simulink model "EDDA_1st"  (R2020a)
settings: Solver=ode45  StartTime=0.0  StopTime=T  RelTol=1e-8
values from neighbouring files (symbols this model uses):
  g = 9.81    [TestingIkRTR.m]    (also in TestingScript.m; TestingScriptRTR.m)
  Kd1 = Kp1/10    (= 100)    [TestingIkRTR.m]    (also in TestingScript.m = 1; TestingScriptRTR.m)
  Kp1 = 1000    [TestingIkRTR.m]    (also in TestingScript.m = 10; TestingScriptRTR.m)
  O1 = 3.1    [TestingScript.m]
  O2 = 9.5    [TestingScript.m]
  O3 = 0.24    [TestingScript.m]
  O4 = 0.77    [TestingScript.m]
settings Model: Creator=ja  LastModifiedBy=ja

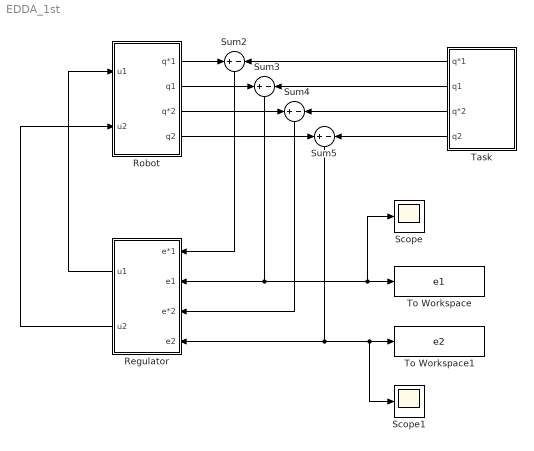
== system EDDA_1st ==
  Regulator : Subsystem
  Robot : Subsystem
  Scope : Scope
  Scope1 : Scope
  Sum{2..5} (4 alike) : Sum  Inputs=+-
  Task : Subsystem
  To Workspace : ToWorkspace  VariableName=e1  SampleTime=-1
  To Workspace1 : ToWorkspace  VariableName=e2  SampleTime=-1
  wires:
  Sum4/1 -> Regulator/3(e*2)
  Sum3/1 -> Regulator/2(e1), Scope/1, To Workspace/1
  Sum2/1 -> Regulator/1(e*1)
  Robot/3(q*2) -> Sum4/1
  Robot/4(q2) -> Sum5/1
  Task/1(q*1) -> Sum2/2
  Sum5/1 -> Regulator/4(e2), Scope1/1, To Workspace1/1
  Robot/2(q1) -> Sum3/1
  Task/2(q1) -> Sum3/2
  Regulator/1(" u1") -> Robot/1(u1)
  Task/4(q2) -> Sum5/2
  Regulator/2(u2) -> Robot/2(u2)
  Robot/1(q*1) -> Sum2/1
  Task/3(q*2) -> Sum4/2

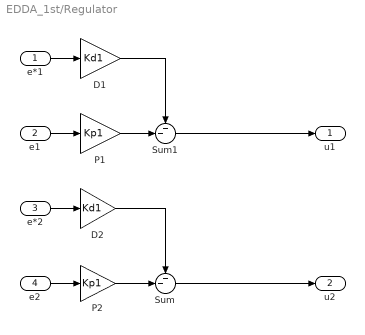
== system EDDA_1st/Regulator ==
  e*1 : Inport
  e1 : Inport  Port=2
  e*2 : Inport  Port=3
  e2 : Inport  Port=4
  D1 : Gain  Gain=Kd1
  D2 : Gain  Gain=Kd1
  P1 : Gain  Gain=Kp1
  P2 : Gain  Gain=Kp1
  Sum : Sum  Inputs=--|
  Sum1 : Sum  Inputs=--|
  " u1" : Outport
  u2 : Outport  Port=2
  wires:
  e2/1 -> P2/1
  Sum/1 -> u2/1
  e*2/1 -> D2/1
  e1/1 -> P1/1
  Sum1/1 -> " u1"/1
  e*1/1 -> D1/1
  D1/1 -> Sum1/1
  P1/1 -> Sum1/2
  D2/1 -> Sum/1
  P2/1 -> Sum/2

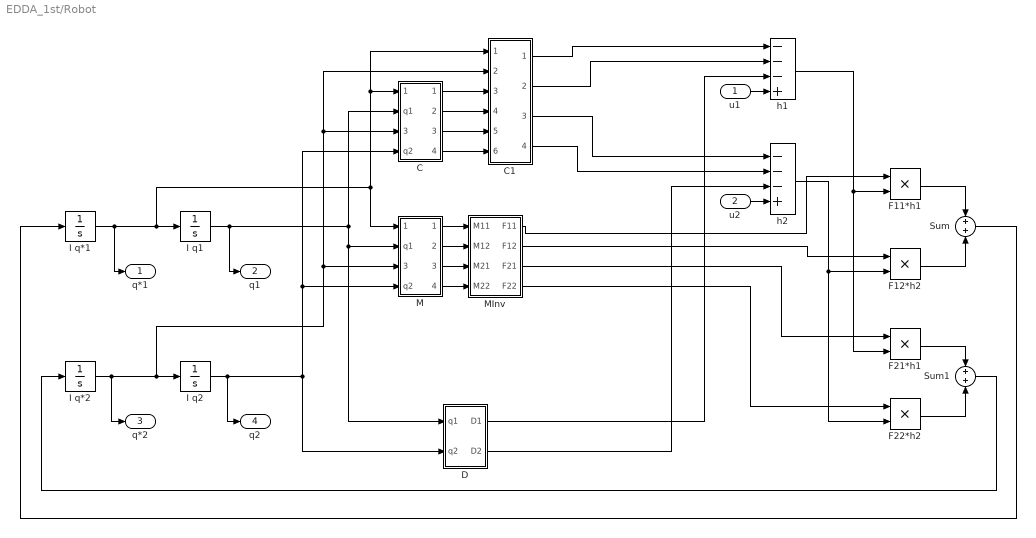
== system EDDA_1st/Robot ==
  u1 : Inport
  u2 : Inport  Port=2
  C : Subsystem
  C1 : Subsystem
  D : Subsystem
  F11*h1 : Product
  F12*h2 : Product
  F21*h1 : Product
  F22*h2 : Product
  I q*1 : Integrator
  I q*2 : Integrator
  I q1 : Integrator
  I q2 : Integrator
  M : Subsystem
  MInv : MATLAB Function  TreatAsAtomicUnit=on
  Sum : Sum
  Sum1 : Sum
  h1 : Sum  Inputs=---+
  h2 : Sum  Inputs=---+
  q*1 : Outport
  q1 : Outport  Port=2
  q*2 : Outport  Port=3
  q2 : Outport  Port=4
  wires:
  I q2/1 -> q2/1, C/4(q2), M/4(q2), D/2(q2)
  Sum/1 -> I q*1/1
  MInv/1(F11) -> F11*h1/1
  M/4(M22) -> MInv/4(M22)
  D/1(D1) -> h1/3
  I q*1/1 -> q*1/1, I q1/1, C1/1(q*1), C/1(q*1), M/1(q*1)
  Sum1/1 -> I q*2/1
  I q1/1 -> q1/1, D/1(q1), M/2(q1), C/2(q1)
  F22*h2/1 -> Sum1/2
  F11*h1/1 -> Sum/1
  I q*2/1 -> q*2/1, M/3(q*2), C1/2(q*2), C/3(q*2), I q2/1
  M/1(M11) -> MInv/1(M11)
  MInv/4(F22) -> F22*h2/1
  F12*h2/1 -> Sum/2
  M/2(M12) -> MInv/2(M12)
  D/2(D2) -> h2/3
  h2/1 -> F12*h2/2, F22*h2/2
  F21*h1/1 -> Sum1/1
  u2/1 -> h2/4
  MInv/2(F12) -> F12*h2/1
  h1/1 -> F21*h1/2, F11*h1/2
  M/3(M21) -> MInv/3(M21)
  u1/1 -> h1/4
  C/1(C11) -> C1/3(C11)
  C/2(C12) -> C1/4(C12)
  C/3(C21) -> C1/5(C21)
  C/4(C22) -> C1/6(C22)
  C1/4(Out4) -> h2/2
  C1/3(Out3) -> h2/1
  C1/1(Out1) -> h1/1
  C1/2(Out2) -> h1/2
  MInv/3(F21) -> F21*h1/1

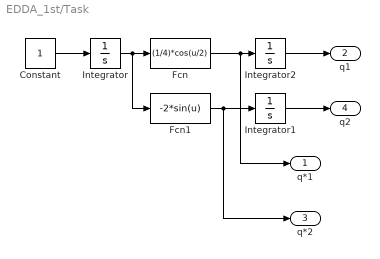
== system EDDA_1st/Task ==
  Constant : Constant
  Fcn : Fcn  Expr=(1/4)*cos(u/2)
  Fcn1 : Fcn  Expr=-2*sin(u)
  Integrator : Integrator
  Integrator1 : Integrator  InitialCondition=2
  Integrator2 : Integrator
  q*1 : Outport
  q1 : Outport  Port=2
  q*2 : Outport  Port=3
  q2 : Outport  Port=4
  wires:
  Constant/1 -> Integrator/1
  Integrator/1 -> Fcn1/1, Fcn/1
  Fcn/1 -> q*1/1, Integrator2/1
  Fcn1/1 -> q*2/1, Integrator1/1
  Integrator2/1 -> q1/1
  Integrator1/1 -> q2/1

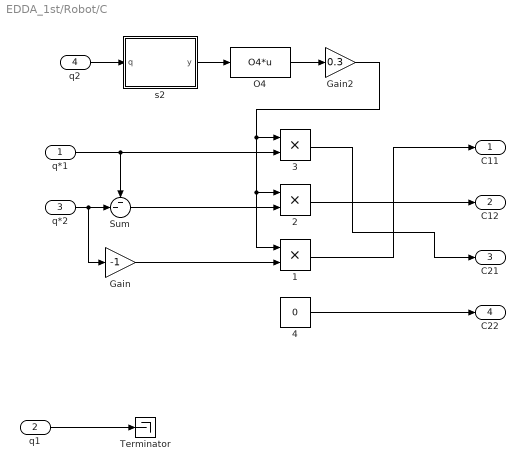
== system EDDA_1st/Robot/C ==
  q*1 : Inport
  q1 : Inport  Port=2
  q*2 : Inport  Port=3
  q2 : Inport  Port=4
  1 : Product
  2 : Product
  3 : Product
  4 : Constant  Value=0
  Gain : Gain  Gain=-1
  Gain2 : Gain  Gain=0.3
  O4 : Fcn  Expr=O4*u
  Sum : Sum  Inputs=--|
  Terminator : Terminator
  s2 : MATLAB Function  TreatAsAtomicUnit=on
  C11 : Outport
  C12 : Outport  Port=2
  C21 : Outport  Port=3
  C22 : Outport  Port=4
  wires:
  q*2/1 -> Gain/1, Sum/2
  q2/1 -> s2/1(q)
  q*1/1 -> 3/2, Sum/1
  s2/1(y) -> O4/1
  O4/1 -> Gain2/1
  Sum/1 -> 2/2
  Gain/1 -> 1/2
  Gain2/1 -> 1/1, 2/1, 3/1
  4/1 -> C22/1
  1/1 -> C11/1
  3/1 -> C21/1
  2/1 -> C12/1
  q1/1 -> Terminator/1

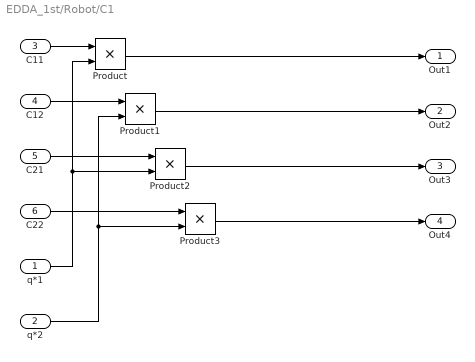
== system EDDA_1st/Robot/C1 ==
  q*1 : Inport
  q*2 : Inport  Port=2
  C11 : Inport  Port=3
  C12 : Inport  Port=4
  C21 : Inport  Port=5
  C22 : Inport  Port=6
  Product{,1..3} (4 alike) : Product
  Out1 : Outport
  Out2 : Outport  Port=2
  Out3 : Outport  Port=3
  Out4 : Outport  Port=4
  wires:
  C11/1 -> Product/1
  C12/1 -> Product1/1
  C21/1 -> Product2/1
  C22/1 -> Product3/1
  q*1/1 -> Product2/2, Product/2
  q*2/1 -> Product3/2, Product1/2
  Product3/1 -> Out4/1
  Product2/1 -> Out3/1
  Product1/1 -> Out2/1
  Product/1 -> Out1/1

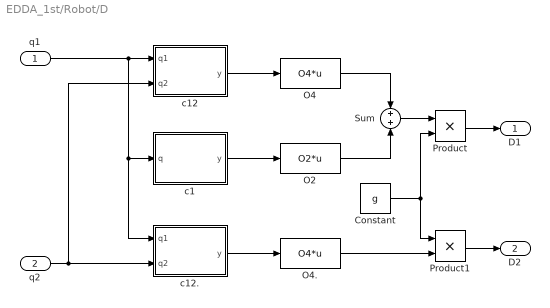
== system EDDA_1st/Robot/D ==
  q1 : Inport
  q2 : Inport  Port=2
  Constant : Constant  Value=g
  O2 : Fcn  Expr=O2*u
  O4 : Fcn  Expr=O4*u
  O4. : Fcn  Expr=O4*u
  Product : Product
  Product1 : Product
  Sum : Sum
  c1 : MATLAB Function  TreatAsAtomicUnit=on
  c12 : MATLAB Function  TreatAsAtomicUnit=on
  c12. : MATLAB Function  TreatAsAtomicUnit=on
  D1 : Outport
  D2 : Outport  Port=2
  wires:
  q1/1 -> c12./1(q1), c1/1(q), c12/1(q1)
  q2/1 -> c12./2(q2), c12/2(q2)
  c12./1(y) -> O4./1
  Product/1 -> D1/1
  Sum/1 -> Product/1
  Product1/1 -> D2/1
  Constant/1 -> Product/2, Product1/1
  O4./1 -> Product1/2
  c12/1(y) -> O4/1
  c1/1(y) -> O2/1
  O2/1 -> Sum/2
  O4/1 -> Sum/1

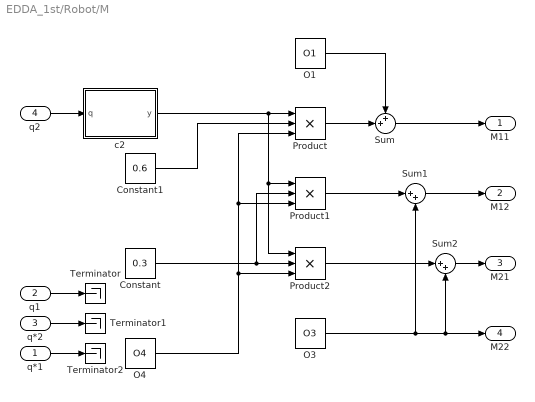
== system EDDA_1st/Robot/M ==
  q*1 : Inport
  q1 : Inport  Port=2
  q*2 : Inport  Port=3
  q2 : Inport  Port=4
  Constant : Constant  Value=0.3
  Constant1 : Constant  Value=0.6
  O1 : Constant  Value=O1
  O3 : Constant  Value=O3
  O4 : Constant  Value=O4
  Product : Product  Inputs=3
  Product1 : Product  Inputs=3
  Product2 : Product  Inputs=3
  Sum : Sum  Inputs=++|
  Sum1 : Sum  Inputs=|++
  Sum2 : Sum  Inputs=|++
  Terminator : Terminator
  Terminator1 : Terminator
  Terminator2 : Terminator
  c2 : MATLAB Function  TreatAsAtomicUnit=on
  M11 : Outport
  M12 : Outport  Port=2
  M21 : Outport  Port=3
  M22 : Outport  Port=4
  wires:
  q2/1 -> c2/1(q)
  c2/1(y) -> Product2/1, Product1/1, Product/1
  Constant1/1 -> Product/2
  Constant/1 -> Product1/2, Product2/2
  q1/1 -> Terminator/1
  q*2/1 -> Terminator1/1
  q*1/1 -> Terminator2/1
  Product/1 -> Sum/2
  Sum/1 -> M11/1
  Sum1/1 -> M12/1
  Sum2/1 -> M21/1
  O3/1 -> Sum1/2, Sum2/2, M22/1
  O1/1 -> Sum/1
  Product1/1 -> Sum1/1
  Product2/1 -> Sum2/1
  O4/1 -> Product/3, Product1/3, Product2/3

== matlab function EDDA_1st/Robot/D/c12. ==
  data: q1 input; y output; q2 input
function y = c12(q1, q2)

y = cos(q1+q2);

== matlab function EDDA_1st/Robot/D/c12 ==
  data: q1 input; y output; q2 input
function y = c12(q1, q2)

y = cos(q1+q2);

== matlab function EDDA_1st/Robot/D/c1 ==
  data: q input; y output
function y = c(q)

y = cos(q);

== matlab function EDDA_1st/Robot/M/c2 ==
  data: q input; y output
function y = c(q)

y = cos(q);

== matlab function EDDA_1st/Robot/C/s2 ==
  data: q input; y output
function y = s(q)

y = sin(q);

== matlab function EDDA_1st/Robot/MInv ==
  data: M11 input; F11 output; M12 input; M21 input; M22 input; F12 output; F21 output; F22 output
function [F11, F12, F21, F22] = c(M11, M12, M21, M22)

M = [M11 M12; M21 M22];
F = inv(M);

F11 = F(1);
F12 = F(2);
F21 = F(3);
F22 = F(4);
